simulink model "UB2_Loesung"  (Simulink 7.5)
settings: Solver=ode3  StartTime=0.0  StopTime=20  FixedStep=0.01  RelTol=1e-3
undefined symbols (not defined in the file): c, d, m
libraries: simulink x1
settings Model: Creator=gaus  LastModifiedBy=M. Geißendörfer
settings DebuggingCC: StrictBusMsg=Warning

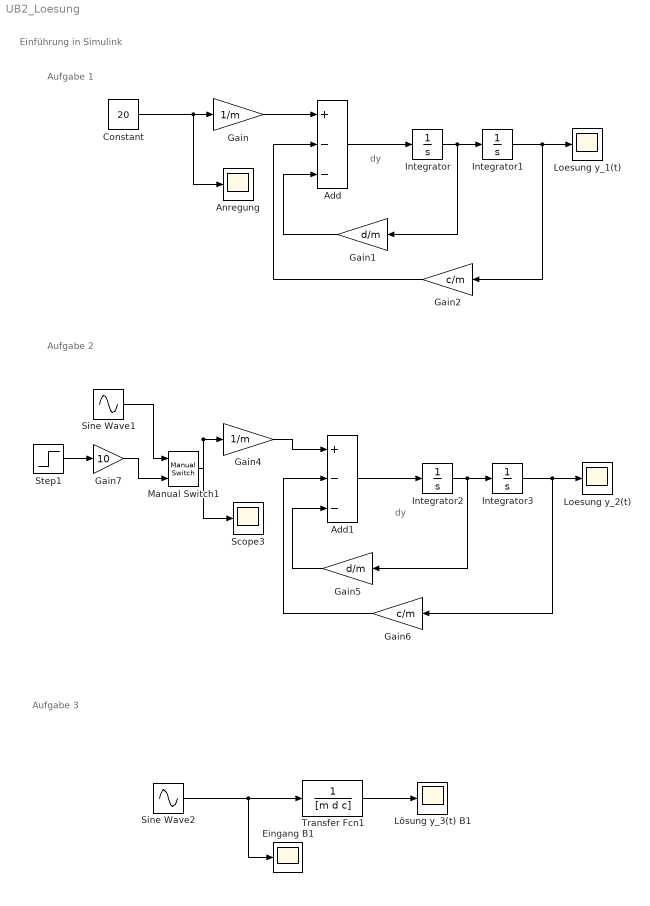
== system UB2_Loesung ==
  note: dy
  note: dy
  note: Aufgabe 2
  note: Aufgabe 1
  note: Aufgabe 3
  note: Einführung in Simulink
  Add : Sum  Inputs=+--  OutDataType=sfix(16)  OutScaling=2^-10
  Add1 : Sum  Inputs=+--  OutDataType=sfix(16)  OutScaling=2^-10
  Anregung : Scope
  Constant : Constant  Value=20  OutDataType=sfix(16)  OutScaling=2^0
  Eingang B1 : Scope
      settings: TimeRange=40  YMin=-1.1  YMax=1.1  SaveName=ScopeData6
  Gain : Gain  Gain=1/m  ParameterDataType=sfix(16)  ParameterScaling=2^0  OutDataType=sfix(16)  OutScaling=2^0
  Gain1 : Gain  Gain=d/m  ParameterDataType=sfix(16)  ParameterScaling=2^0  OutDataType=sfix(16)  OutScaling=2^0
  Gain2 : Gain  Gain=c/m  ParameterDataType=sfix(16)  ParameterScaling=2^0  OutDataType=sfix(16)  OutScaling=2^0
  Gain4 : Gain  Gain=1/m  ParameterDataType=sfix(16)  ParameterScaling=2^0  OutDataType=sfix(16)  OutScaling=2^0
  Gain5 : Gain  Gain=d/m  ParameterDataType=sfix(16)  ParameterScaling=2^0  OutDataType=sfix(16)  OutScaling=2^0
  Gain6 : Gain  Gain=c/m  ParameterDataType=sfix(16)  ParameterScaling=2^0  OutDataType=sfix(16)  OutScaling=2^0
  Gain7 : Gain  Gain=10  ParameterDataType=sfix(16)  ParameterScaling=2^0  OutDataType=sfix(16)  OutScaling=2^0
  Integrator{,1..3} (4 alike) : Integrator
  Loesung y_1(t) : Scope
  Loesung y_2(t) : Scope
      settings: SaveName=ScopeData3
  Lösung y_3(t) B1 : Scope
      settings: YMin=-0.6  YMax=0.6  SaveName=ScopeData7
  Manual Switch1 : simulink/Signal Routing/Manual Switch  SystemSampleTime=-1  sw=1  action=0  varsize=off
  Scope3 : Scope
      settings: SaveName=ScopeData2
  Sine Wave1 : Sin  Amplitude=20  Bias=0  Frequency=2  Phase=0  Samples=10  SampleTime=0  Offset=0
  Sine Wave2 : Sin  Amplitude=20  Bias=0  Frequency=2  Phase=0  Samples=10  SampleTime=0  Offset=0
  Step1 : Step  SampleTime=0
  Transfer Fcn1 : TransferFcn  Denominator=[m d c]
  wires:
  Integrator/1 -> Integrator1/1, Gain1/1
  Gain1/1 -> Add/3
  Add/1 -> Integrator/1
  Integrator1/1 -> Gain2/1, Loesung y_1(t)/1
  Gain/1 -> Add/1
  Gain2/1 -> Add/2
  Constant/1 -> Gain/1, Anregung/1
  Integrator2/1 -> Gain5/1, Integrator3/1
  Gain5/1 -> Add1/3
  Add1/1 -> Integrator2/1
  Integrator3/1 -> Loesung y_2(t)/1, Gain6/1
  Gain4/1 -> Add1/1
  Gain6/1 -> Add1/2
  Manual Switch1/1 -> Scope3/1, Gain4/1
  Sine Wave1/1 -> Manual Switch1/1
  Step1/1 -> Gain7/1
  Gain7/1 -> Manual Switch1/2
  Transfer Fcn1/1 -> Lösung y_3(t) B1/1
  Sine Wave2/1 -> Transfer Fcn1/1, Eingang B1/1
